simulink model "microgrid"  (R2021a)
settings: Solver=ode23t  StartTime=0.0  StopTime=24*60*60  FixedStep=1/(1000)  MaxStep=60  RelTol=1e-4
PreLoadFcn:
  | load('solar_load_data_24h.mat')
undefined symbols (not defined in the file or in its folder): Angle, Cp_max, J_t, K_t, lambda_opt, Magnitude, rho, sigbuilder_block
libraries: fl_lib x14, ee_lib x12, spsCurrentMeasurementLib x7, spsSeriesRLCBranchLib x6, spsControlledCurrentSourceLib x5, spsGroundLib x5, nesl_utility x3, spsSeriesRLCLoadLib x3, simulink x2, spsVoltageMeasurementLib x2, spsThreePhaseTransformerTwoWindingsLib x1, spsLinearTransformerLib x1
(part 2 of 2)

== system microgrid/Battery1/Storage1 ==
  I_RMS : Inport
  Add : Sum  Inputs=+-
  Constant : Constant  Value=5*0.2*3600
  Constant1 : Constant  Value=0.5
  Gain : Gain  Gain=1/3600
  Gain3 : Gain  Gain=1/(5*3600)
  Gain8 : Gain  Gain=200
  Integrator : Integrator
  Integrator1 : Integrator  InitialConditionSource=external
  Battery_Ah : Outport  VectorParamsAs1DForOutWhenUnconnected=off
  Battery_SOC : Outport  Port=2  VectorParamsAs1DForOutWhenUnconnected=off
  wires:
  Integrator/1 -> Gain/1
  Integrator1/1 -> Gain3/1
  Gain3/1 -> Add/2
  Constant1/1 -> Add/1
  Add/1 -> Gain8/1
  Constant/1 -> Integrator1/2
  I_RMS/1 -> Integrator/1, Integrator1/1
  Gain/1 -> Battery_Ah/1
  Gain8/1 -> Battery_SOC/1

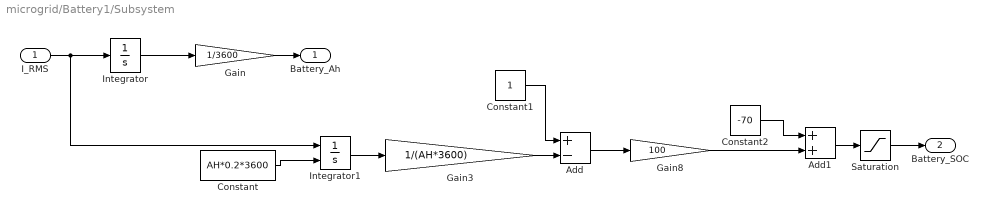
== system microgrid/Battery1/Subsystem ==
  I_RMS : Inport
  Add : Sum  Inputs=+-
  Add1 : Sum
  Constant : Constant  Value=AH*0.2*3600
  Constant1 : Constant
  Constant2 : Constant  Value=-70
  Gain : Gain  Gain=1/3600
  Gain3 : Gain  Gain=1/(AH*3600)
  Gain8 : Gain  Gain=100
  Integrator : Integrator
  Integrator1 : Integrator  InitialConditionSource=external
  Saturation : Saturate  UpperLimit=100  LowerLimit=0
  Battery_Ah : Outport  VectorParamsAs1DForOutWhenUnconnected=off
  Battery_SOC : Outport  Port=2  VectorParamsAs1DForOutWhenUnconnected=off
  wires:
  Integrator/1 -> Gain/1
  Integrator1/1 -> Gain3/1
  Gain3/1 -> Add/2
  Constant1/1 -> Add/1
  Add/1 -> Gain8/1
  Constant/1 -> Integrator1/2
  I_RMS/1 -> Integrator/1, Integrator1/1
  Gain/1 -> Battery_Ah/1
  Saturation/1 -> Battery_SOC/1
  Add1/1 -> Saturation/1
  Gain8/1 -> Add1/2
  Constant2/1 -> Add1/1

== system microgrid/PV/Module1 ==
  Diode2 : fl_lib/Electrical/Electrical Elements/Diode  Vf=0.6 V  Ron=0.3 Ohm  Goff=1e-8 1/Ohm  i_specify=off  i_priority=None  i=0 A  i_nominal_specify=off  i_nominal_unit=A  i_nominal_value=1  v_specify=off  v_priority=None  v=0 V  v_nominal_specify=off  v_nominal_unit=V  v_nominal_value=1
  Diode3 : fl_lib/Electrical/Electrical Elements/Diode  Vf=0.6 V  Ron=0.3 Ohm  Goff=1e-8 1/Ohm  i_specify=off  i_priority=None  i=0 A  i_nominal_specify=off  i_nominal_unit=A  i_nominal_value=1  v_specify=off  v_priority=None  v=0 V  v_nominal_specify=off  v_nominal_unit=V  v_nominal_value=1
  Diode4 : fl_lib/Electrical/Electrical Elements/Diode  Vf=0.6 V  Ron=0.3 Ohm  Goff=1e-8 1/Ohm  i_specify=off  i_priority=None  i=0 A  i_nominal_specify=off  i_nominal_unit=A  i_nominal_value=1  v_specify=off  v_priority=None  v=0 V  v_nominal_specify=off  v_nominal_unit=V  v_nominal_value=1
  Solar Cell : ee_lib/Sources/Solar Cell  prm=1  Isc=3 A  Voc=3 V  Is=1e-6 A  Is2=0 A  Iph=7.34 A  Ir0=1000 W/m^2  ec=1.5  N2=2  Rs=0 Ohm  Rp=inf Ohm  N_series=1  TIPH1=0 1/K  EG=1.11 eV  TXIS1=3  TXIS2=3  TRS1=0  TRP1=0  Tmeas=25 degC  TFIXED=25 degC  thermal_mass=100 J/K  initial_temperature=25 degC
      settings: SourceProductBaseCode=PS
  Solar Cell1 : ee_lib/Sources/Solar Cell  prm=1  Isc=3 A  Voc=3 V  Is=1e-6 A  Is2=0 A  Iph=7.34 A  Ir0=1000 W/m^2  ec=1.5  N2=2  Rs=0 Ohm  Rp=inf Ohm  N_series=1  TIPH1=0 1/K  EG=1.11 eV  TXIS1=3  TXIS2=3  TRS1=0  TRP1=0  Tmeas=25 degC  TFIXED=25 degC  thermal_mass=100 J/K  initial_temperature=25 degC
      settings: SourceProductBaseCode=PS
  Solar Cell2 : ee_lib/Sources/Solar Cell  prm=1  Isc=3 A  Voc=3 V  Is=1e-6 A  Is2=0 A  Iph=7.34 A  Ir0=1000 W/m^2  ec=1.5  N2=2  Rs=0 Ohm  Rp=inf Ohm  N_series=1  TIPH1=0 1/K  EG=1.11 eV  TXIS1=3  TXIS2=3  TRS1=0  TRP1=0  Tmeas=25 degC  TFIXED=25 degC  thermal_mass=100 J/K  initial_temperature=25 degC
      settings: SourceProductBaseCode=PS
  constant : PMIOPort  Side=Left
  positive : PMIOPort  Port=2  Side=Left
  negative : PMIOPort  Port=3  Side=Right
  connections:
  Diode2/RConn1 -- Solar Cell2/LConn2 -- positive/RConn1
  Diode2/LConn1 -- Solar Cell2/RConn1 -- Diode3/RConn1 -- Solar Cell1/LConn2
  Solar Cell1/RConn1 -- Diode3/LConn1 -- Diode4/RConn1 -- Solar Cell/LConn2
  negative/RConn1 -- Diode4/LConn1 -- Solar Cell/RConn1
  Solar Cell2/LConn1 -- constant/RConn1 -- Solar Cell/LConn1 -- Solar Cell1/LConn1

== system microgrid/PV/Module2 ==
  Diode2 : fl_lib/Electrical/Electrical Elements/Diode  Vf=0.6 V  Ron=0.3 Ohm  Goff=1e-8 1/Ohm  i_specify=off  i_priority=None  i=0 A  i_nominal_specify=off  i_nominal_unit=A  i_nominal_value=1  v_specify=off  v_priority=None  v=0 V  v_nominal_specify=off  v_nominal_unit=V  v_nominal_value=1
  Diode3 : fl_lib/Electrical/Electrical Elements/Diode  Vf=0.6 V  Ron=0.3 Ohm  Goff=1e-8 1/Ohm  i_specify=off  i_priority=None  i=0 A  i_nominal_specify=off  i_nominal_unit=A  i_nominal_value=1  v_specify=off  v_priority=None  v=0 V  v_nominal_specify=off  v_nominal_unit=V  v_nominal_value=1
  Diode4 : fl_lib/Electrical/Electrical Elements/Diode  Vf=0.6 V  Ron=0.3 Ohm  Goff=1e-8 1/Ohm  i_specify=off  i_priority=None  i=0 A  i_nominal_specify=off  i_nominal_unit=A  i_nominal_value=1  v_specify=off  v_priority=None  v=0 V  v_nominal_specify=off  v_nominal_unit=V  v_nominal_value=1
  Solar Cell : ee_lib/Sources/Solar Cell  prm=1  Isc=3 A  Voc=3 V  Is=1e-6 A  Is2=0 A  Iph=7.34 A  Ir0=1000 W/m^2  ec=1.5  N2=2  Rs=0 Ohm  Rp=inf Ohm  N_series=1  TIPH1=0 1/K  EG=1.11 eV  TXIS1=3  TXIS2=3  TRS1=0  TRP1=0  Tmeas=25 degC  TFIXED=25 degC  thermal_mass=100 J/K  initial_temperature=25 degC
      settings: SourceProductBaseCode=PS
  Solar Cell1 : ee_lib/Sources/Solar Cell  prm=1  Isc=3 A  Voc=3 V  Is=1e-6 A  Is2=0 A  Iph=7.34 A  Ir0=1000 W/m^2  ec=1.5  N2=2  Rs=0 Ohm  Rp=inf Ohm  N_series=1  TIPH1=0 1/K  EG=1.11 eV  TXIS1=3  TXIS2=3  TRS1=0  TRP1=0  Tmeas=25 degC  TFIXED=25 degC  thermal_mass=100 J/K  initial_temperature=25 degC
      settings: SourceProductBaseCode=PS
  Solar Cell2 : ee_lib/Sources/Solar Cell  prm=1  Isc=3 A  Voc=3 V  Is=1e-6 A  Is2=0 A  Iph=7.34 A  Ir0=1000 W/m^2  ec=1.5  N2=2  Rs=0 Ohm  Rp=inf Ohm  N_series=1  TIPH1=0 1/K  EG=1.11 eV  TXIS1=3  TXIS2=3  TRS1=0  TRP1=0  Tmeas=25 degC  TFIXED=25 degC  thermal_mass=100 J/K  initial_temperature=25 degC
      settings: SourceProductBaseCode=PS
  constant : PMIOPort  Side=Left
  positive : PMIOPort  Port=2  Side=Left
  negative : PMIOPort  Port=3  Side=Right
  connections:
  Diode2/RConn1 -- Solar Cell2/LConn2 -- positive/RConn1
  Diode2/LConn1 -- Solar Cell2/RConn1 -- Diode3/RConn1 -- Solar Cell1/LConn2
  Solar Cell1/RConn1 -- Diode3/LConn1 -- Diode4/RConn1 -- Solar Cell/LConn2
  negative/RConn1 -- Diode4/LConn1 -- Solar Cell/RConn1
  Solar Cell2/LConn1 -- constant/RConn1 -- Solar Cell/LConn1 -- Solar Cell1/LConn1

== system microgrid/PV/Module3 ==
  Diode2 : fl_lib/Electrical/Electrical Elements/Diode  Vf=0.6 V  Ron=0.3 Ohm  Goff=1e-8 1/Ohm  i_specify=off  i_priority=None  i=0 A  i_nominal_specify=off  i_nominal_unit=A  i_nominal_value=1  v_specify=off  v_priority=None  v=0 V  v_nominal_specify=off  v_nominal_unit=V  v_nominal_value=1
  Diode3 : fl_lib/Electrical/Electrical Elements/Diode  Vf=0.6 V  Ron=0.3 Ohm  Goff=1e-8 1/Ohm  i_specify=off  i_priority=None  i=0 A  i_nominal_specify=off  i_nominal_unit=A  i_nominal_value=1  v_specify=off  v_priority=None  v=0 V  v_nominal_specify=off  v_nominal_unit=V  v_nominal_value=1
  Diode4 : fl_lib/Electrical/Electrical Elements/Diode  Vf=0.6 V  Ron=0.3 Ohm  Goff=1e-8 1/Ohm  i_specify=off  i_priority=None  i=0 A  i_nominal_specify=off  i_nominal_unit=A  i_nominal_value=1  v_specify=off  v_priority=None  v=0 V  v_nominal_specify=off  v_nominal_unit=V  v_nominal_value=1
  Solar Cell : ee_lib/Sources/Solar Cell  prm=1  Isc=3 A  Voc=3 V  Is=1e-6 A  Is2=0 A  Iph=7.34 A  Ir0=1000 W/m^2  ec=1.5  N2=2  Rs=0 Ohm  Rp=inf Ohm  N_series=1  TIPH1=0 1/K  EG=1.11 eV  TXIS1=3  TXIS2=3  TRS1=0  TRP1=0  Tmeas=25 degC  TFIXED=25 degC  thermal_mass=100 J/K  initial_temperature=25 degC
      settings: SourceProductBaseCode=PS
  Solar Cell1 : ee_lib/Sources/Solar Cell  prm=1  Isc=3 A  Voc=3 V  Is=1e-6 A  Is2=0 A  Iph=7.34 A  Ir0=1000 W/m^2  ec=1.5  N2=2  Rs=0 Ohm  Rp=inf Ohm  N_series=1  TIPH1=0 1/K  EG=1.11 eV  TXIS1=3  TXIS2=3  TRS1=0  TRP1=0  Tmeas=25 degC  TFIXED=25 degC  thermal_mass=100 J/K  initial_temperature=25 degC
      settings: SourceProductBaseCode=PS
  Solar Cell2 : ee_lib/Sources/Solar Cell  prm=1  Isc=3 A  Voc=3 V  Is=1e-6 A  Is2=0 A  Iph=7.34 A  Ir0=1000 W/m^2  ec=1.5  N2=2  Rs=0 Ohm  Rp=inf Ohm  N_series=1  TIPH1=0 1/K  EG=1.11 eV  TXIS1=3  TXIS2=3  TRS1=0  TRP1=0  Tmeas=25 degC  TFIXED=25 degC  thermal_mass=100 J/K  initial_temperature=25 degC
      settings: SourceProductBaseCode=PS
  constant : PMIOPort  Side=Left
  positive : PMIOPort  Port=2  Side=Left
  negative : PMIOPort  Port=3  Side=Right
  connections:
  Diode2/RConn1 -- Solar Cell2/LConn2 -- positive/RConn1
  Diode2/LConn1 -- Solar Cell2/RConn1 -- Diode3/RConn1 -- Solar Cell1/LConn2
  Solar Cell1/RConn1 -- Diode3/LConn1 -- Diode4/RConn1 -- Solar Cell/LConn2
  negative/RConn1 -- Diode4/LConn1 -- Solar Cell/RConn1
  Solar Cell2/LConn1 -- constant/RConn1 -- Solar Cell/LConn1 -- Solar Cell1/LConn1

== system microgrid/Scenario/Signal Builder ==
  Demux : Demux  Tag=STV Demux  Outputs=1
      settings: DisplayOption=none
  FromWs : FromWorkspace  Tag=STV FromWs  VariableName=tuvar
      SigBuilderData=|
      | common.afterFinalStr = 'Extrapolate'
      | common.sampleTime = 0
      | dataSet.timeRange = [0 84600]
      | dataSet.name = 'Sheet1'
      | sbobj.Groups.Name = 'Sheet1'
      | sbobj.Groups.Signals.Name = 'demand(MW)'
      | sbobj.Groups.Signals.XData = [0 1800 3600 5400 7200 9000 10800 12600 14400 16200 18000 19800 21600 23400 25200 27000 28800 30600 32400 34200 36000 37800 39600 41400 43200 45000 46800 48600 50400 52200 54000 55800 57600 59400 61200 63000 64800 66600 68400 70200 72000 73800 75600 77400 79200 81000 82800 84600]
      | sbobj.Groups.Signals.YData = [4.235 4.305 3.745 2.555 2.31 2.485 2.38 1.855 2.59 4.025 12.18 19.18 17.92 6.685 3.71 3.78 4.165 4.305 3.815 2.555 18.305 7.525 6.545 7.91 4.9 11.27 21.805 10.115 16.59 3.71 4.41 4.515 4.41 3.605 5.635 7.56 11.305 17.99 28.77 21.245 15.61 14.315 16.1 10.43 8.645 4.41 3.78 5.355]
      | sbobj.Groups.TimeRange = [0 84600]
  demand(MW) : Outport  Tag=STV Outport
  wires:
  Demux/1 -> demand(MW)/1
  FromWs/1 -> Demux/1

== system microgrid/Scenario/Signal Builder1 ==
  Demux : Demux  Tag=STV Demux  Outputs=1
      settings: DisplayOption=none
  FromWs : FromWorkspace  Tag=STV FromWs  VariableName=tuvar
      SigBuilderData=|
      | common.afterFinalStr = 'Extrapolate'
      | common.sampleTime = 0
      | dataSet.timeRange = [0 86340]
      | dataSet.name = 'Sheet1'
      | sbobj.Groups.Name = 'Sheet1'
      | sbobj.Groups.Signals.Name = 'DNI_Avg'
      | sbobj.Groups.Signals.XData = [0 60 120 180 240 300 360 420 480 540 600 660 ... (1440 elements, 1x1440)]
      | sbobj.Groups.Signals.YData = [-2.093828 0.820727 -1.83532 -1.790075 -2.694803 -2.151961 1.518648 -0.6850063 1.628504 0.8336399 -0.05816128 0.05816069 ... (1440 elements, 1x1440)]
      | sbobj.Groups.TimeRange = [0 84600]
  DNI_Avg : Outport  Tag=STV Outport
  wires:
  Demux/1 -> DNI_Avg/1
  FromWs/1 -> Demux/1

== system microgrid/Scenario/Signal Builder2 ==
  Demux : Demux  Tag=STV Demux  Outputs=1
      settings: DisplayOption=none
  FromWs : FromWorkspace  Tag=STV FromWs  VariableName=tuvar
      SigBuilderData=|
      | common.afterFinalStr = 'Extrapolate'
      | common.sampleTime = 0
      | dataSet.timeRange = [0 86340]
      | dataSet.name = 'Sheet1'
      | sbobj.Groups.Name = 'Sheet1'
      | sbobj.Groups.Signals.Name = 'DNI_Avg'
      | sbobj.Groups.Signals.XData = [0 60 120 180 240 300 360 420 480 540 600 660 ... (1440 elements, 1x1440)]
      | sbobj.Groups.Signals.YData = [-2.093828 0.820727 -1.83532 -1.790075 -2.694803 -2.151961 1.518648 -0.6850063 1.628504 0.8336399 -0.05816128 0.05816069 ... (1440 elements, 1x1440)]
      | sbobj.Groups.TimeRange = [0 86340]
  DNI_Avg : Outport  Tag=STV Outport
  wires:
  Demux/1 -> DNI_Avg/1
  FromWs/1 -> Demux/1

== system microgrid/Scenario/Signal Builder3 ==
  Demux : Demux  Tag=STV Demux  Outputs=1
      settings: DisplayOption=none
  FromWs : FromWorkspace  Tag=STV FromWs  VariableName=tuvar
      SigBuilderData=|
      | common.afterFinalStr = 'Extrapolate'
      | common.sampleTime = 0
      | dataSet.timeRange = [0 86400]
      | dataSet.name = 'Sheet1'
      | sbobj.Groups.Name = 'Sheet1'
      | sbobj.Groups.Signals.Name = 'wind(km/h)'
      | sbobj.Groups.Signals.XData = [0 60 120 180 240 300 360 420 480 540 600 660 ... (1441 elements, 1x1441)]
      | sbobj.Groups.Signals.YData = [23.8995 23.9313 22.97281 18.62791 18.81602 18.57941 17.58444 22.33634 21.24497 21.8146 9.291438 10.73356 ... (1441 elements, 1x1441)]
      | sbobj.Groups.TimeRange = [0 84600]
  wind(km/h) : Outport  Tag=STV Outport
  wires:
  Demux/1 -> wind(km/h)/1
  FromWs/1 -> Demux/1

== system microgrid/Scopes/Active & Reactive Power (Phasor Type) ==
  V : Inport
  I : Inport  Port=2
  Complex to Real-Imag : ComplexToRealImag
  K : Gain  Gain=1/2  SaturateOnIntegerOverflow=on  OutDataTypeStr=Inherit: Same as input  ParamDataTypeStr=Inherit: Same as input
  Math Function : Math  Operator=conj  SignedPower=on  SaturateOnIntegerOverflow=on
  Mux : Mux  Inputs=2
  Product2 : Product  InputSameDT=on  SaturateOnIntegerOverflow=on  OutDataTypeStr=Inherit: Same as first input
  PQ : Outport  VectorParamsAs1DForOutWhenUnconnected=off
  wires:
  Mux/1 -> PQ/1
  Complex to Real-Imag/2 -> Mux/2
  Complex to Real-Imag/1 -> Mux/1
  V/1 -> Product2/1
  Math Function/1 -> Product2/2
  Product2/1 -> K/1
  K/1 -> Complex to Real-Imag/1
  I/1 -> Math Function/1

== system microgrid/Scopes/Active & Reactive Power (Phasor Type)1 ==
  V : Inport
  I : Inport  Port=2
  Complex to Real-Imag : ComplexToRealImag
  K : Gain  Gain=1/2  SaturateOnIntegerOverflow=on  OutDataTypeStr=Inherit: Same as input  ParamDataTypeStr=Inherit: Same as input
  Math Function : Math  Operator=conj  SignedPower=on  SaturateOnIntegerOverflow=on
  Mux : Mux  Inputs=2
  Product2 : Product  InputSameDT=on  SaturateOnIntegerOverflow=on  OutDataTypeStr=Inherit: Same as first input
  PQ : Outport  VectorParamsAs1DForOutWhenUnconnected=off
  wires:
  Mux/1 -> PQ/1
  Complex to Real-Imag/2 -> Mux/2
  Complex to Real-Imag/1 -> Mux/1
  V/1 -> Product2/1
  Math Function/1 -> Product2/2
  Product2/1 -> K/1
  K/1 -> Complex to Real-Imag/1
  I/1 -> Math Function/1

== system microgrid/Scopes/Active & Reactive Power (Phasor Type)2 ==
  V : Inport
  I : Inport  Port=2
  Complex to Real-Imag : ComplexToRealImag
  K : Gain  Gain=1/2  SaturateOnIntegerOverflow=on  OutDataTypeStr=Inherit: Same as input  ParamDataTypeStr=Inherit: Same as input
  Math Function : Math  Operator=conj  SignedPower=on  SaturateOnIntegerOverflow=on
  Mux : Mux  Inputs=2
  Product2 : Product  InputSameDT=on  SaturateOnIntegerOverflow=on  OutDataTypeStr=Inherit: Same as first input
  PQ : Outport  VectorParamsAs1DForOutWhenUnconnected=off
  wires:
  Mux/1 -> PQ/1
  Complex to Real-Imag/2 -> Mux/2
  Complex to Real-Imag/1 -> Mux/1
  V/1 -> Product2/1
  Math Function/1 -> Product2/2
  Product2/1 -> K/1
  K/1 -> Complex to Real-Imag/1
  I/1 -> Math Function/1

== system microgrid/Scopes/Active & Reactive Power (Phasor Type)3 ==
  V : Inport
  I : Inport  Port=2
  Complex to Real-Imag : ComplexToRealImag
  K : Gain  Gain=1/2  SaturateOnIntegerOverflow=on  OutDataTypeStr=Inherit: Same as input  ParamDataTypeStr=Inherit: Same as input
  Math Function : Math  Operator=conj  SignedPower=on  SaturateOnIntegerOverflow=on
  Mux : Mux  Inputs=2
  Product2 : Product  InputSameDT=on  SaturateOnIntegerOverflow=on  OutDataTypeStr=Inherit: Same as first input
  PQ : Outport  VectorParamsAs1DForOutWhenUnconnected=off
  wires:
  Mux/1 -> PQ/1
  Complex to Real-Imag/2 -> Mux/2
  Complex to Real-Imag/1 -> Mux/1
  V/1 -> Product2/1
  Math Function/1 -> Product2/2
  Product2/1 -> K/1
  K/1 -> Complex to Real-Imag/1
  I/1 -> Math Function/1

== system microgrid/Scopes/Active & Reactive Power (Phasor Type)4 ==
  V : Inport
  I : Inport  Port=2
  Complex to Real-Imag : ComplexToRealImag
  K : Gain  Gain=1/2  SaturateOnIntegerOverflow=on  OutDataTypeStr=Inherit: Same as input  ParamDataTypeStr=Inherit: Same as input
  Math Function : Math  Operator=conj  SignedPower=on  SaturateOnIntegerOverflow=on
  Mux : Mux  Inputs=2
  Product2 : Product  InputSameDT=on  SaturateOnIntegerOverflow=on  OutDataTypeStr=Inherit: Same as first input
  PQ : Outport  VectorParamsAs1DForOutWhenUnconnected=off
  wires:
  Mux/1 -> PQ/1
  Complex to Real-Imag/2 -> Mux/2
  Complex to Real-Imag/1 -> Mux/1
  V/1 -> Product2/1
  Math Function/1 -> Product2/2
  Product2/1 -> K/1
  K/1 -> Complex to Real-Imag/1
  I/1 -> Math Function/1

== system microgrid/Scopes/Active & Reactive Power (Phasor Type)5 ==
  V : Inport
  I : Inport  Port=2
  Complex to Real-Imag : ComplexToRealImag
  K : Gain  Gain=1/2  SaturateOnIntegerOverflow=on  OutDataTypeStr=Inherit: Same as input  ParamDataTypeStr=Inherit: Same as input
  Math Function : Math  Operator=conj  SignedPower=on  SaturateOnIntegerOverflow=on
  Mux : Mux  Inputs=2
  Product2 : Product  InputSameDT=on  SaturateOnIntegerOverflow=on  OutDataTypeStr=Inherit: Same as first input
  PQ : Outport  VectorParamsAs1DForOutWhenUnconnected=off
  wires:
  Mux/1 -> PQ/1
  Complex to Real-Imag/2 -> Mux/2
  Complex to Real-Imag/1 -> Mux/1
  V/1 -> Product2/1
  Math Function/1 -> Product2/2
  Product2/1 -> K/1
  K/1 -> Complex to Real-Imag/1
  I/1 -> Math Function/1

== system microgrid/Subsystem2/Gear Box ==
  T_a : Inport
  T_g : Inport  Port=2
  Add : Sum  Inputs=+-
  Gain : Gain  Gain=1/J_t
  Gain1 : Gain  Gain=-K_t/J_t
  Integrator : Integrator  InitialCondition=1.5
  Sum : Sum  Inputs=|++
  omg_r : Outport
  wires:
  T_g/1 -> Add/2
  T_a/1 -> Add/1
  Add/1 -> Gain/1
  Integrator/1 -> Gain1/1, omg_r/1
  Gain1/1 -> Sum/2
  Sum/1 -> Integrator/1
  Gain/1 -> Sum/1

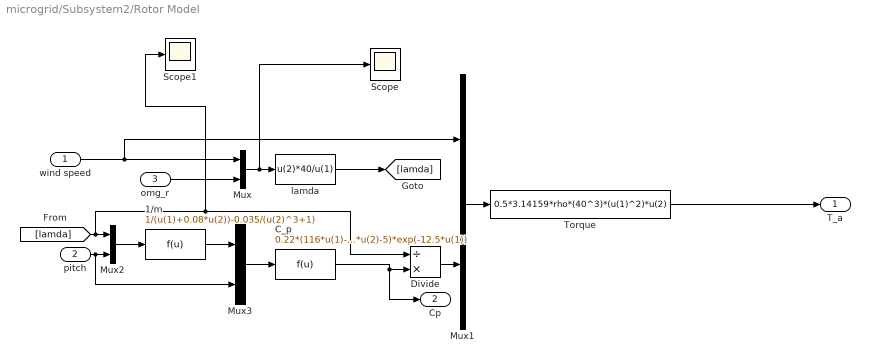
== system microgrid/Subsystem2/Rotor Model ==
  wind speed : Inport
  pitch : Inport  Port=2
  omg_r : Inport  Port=3
  1/m : Fcn  Expr=1/(u(1)+0.08*u(2))-0.035/(u(2)^3+1)
  C_p : Fcn  Expr=0.22*(116*u(1)-0.4*u(2)-5)*exp(-12.5*u(1))
  Divide : Product  Inputs=/*
  Mux{,1..3} (4 alike) : Mux  Inputs=2
  Scope : Scope
  Scope1 : Scope
  Torque : Fcn  Expr=0.5*3.14159*rho*(40^3)*(u(1)^2)*u(2)
  lamda : Fcn  Expr=u(2)*40/u(1)
  T_a : Outport
  Cp : Outport  Port=2
  wires:
  omg_r/1 -> Mux/2
  Mux/1 -> Scope/1, lamda/1
  Mux1/1 -> Torque/1
  lamda/1 -> [lamda]
  [lamda] -> Scope1/1, Divide/1, Mux2/1
  pitch/1 -> Mux3/2, Mux2/2
  Mux2/1 -> 1/m/1
  1/m/1 -> Mux3/1
  C_p/1 -> Divide/2, Cp/1
  Mux3/1 -> C_p/1
  Divide/1 -> Mux1/2
  wind speed/1 -> Mux/1, Mux1/1
  Torque/1 -> T_a/1

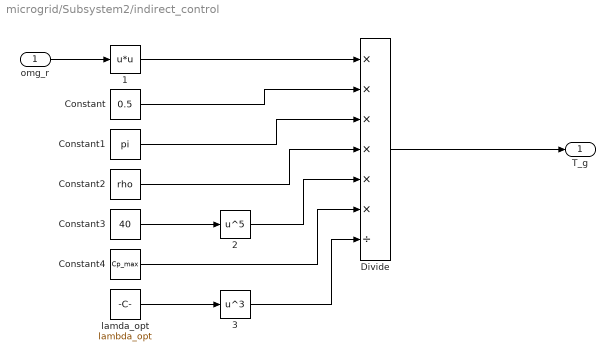
== system microgrid/Subsystem2/indirect_control ==
  omg_r : Inport
  1 : Fcn  Expr=u*u
  2 : Fcn  Expr=u^5
  3 : Fcn  Expr=u^3
  Constant : Constant  Value=0.5
  Constant1 : Constant  Value=pi
  Constant2 : Constant  Value=rho
  Constant3 : Constant  Value=40
  Constant4 : Constant  Value=Cp_max
  Divide : Product  Inputs=******/
  lamda_opt : Constant  Value=lambda_opt
  T_g : Outport
  wires:
  omg_r/1 -> 1/1
  Constant3/1 -> 2/1
  lamda_opt/1 -> 3/1
  1/1 -> Divide/1
  Constant/1 -> Divide/2
  Constant1/1 -> Divide/3
  Constant2/1 -> Divide/4
  2/1 -> Divide/5
  Constant4/1 -> Divide/6
  3/1 -> Divide/7
  Divide/1 -> T_g/1

== system microgrid/Battery1/Battery_Control/Active & Reactive Power (Phasor Type) ==
  V : Inport
  I : Inport  Port=2
  Complex to Real-Imag : ComplexToRealImag
  K : Gain  Gain=1/2  SaturateOnIntegerOverflow=on  OutDataTypeStr=Inherit: Same as input  ParamDataTypeStr=Inherit: Same as input
  Math Function : Math  Operator=conj  SignedPower=on  SaturateOnIntegerOverflow=on
  Mux : Mux  Inputs=2
  Product2 : Product  InputSameDT=on  SaturateOnIntegerOverflow=on  OutDataTypeStr=Inherit: Same as first input
  PQ : Outport  VectorParamsAs1DForOutWhenUnconnected=off
  wires:
  Mux/1 -> PQ/1
  Complex to Real-Imag/2 -> Mux/2
  Complex to Real-Imag/1 -> Mux/1
  V/1 -> Product2/1
  Math Function/1 -> Product2/2
  Product2/1 -> K/1
  K/1 -> Complex to Real-Imag/1
  I/1 -> Math Function/1
